simulink model "oneFingerGACTest2015a"  (R2015a)
settings: Solver=ode45  StartTime=0.0  StopTime=3  RelTol=1e-3
settings Model: CovModelRefEnable=off  Creator=Ricardo  LastModifiedBy=Ricardo
settings DataIOCC: SaveFormat=Dataset
settings HardwareCC: ProdBitPerPointer=64  ProdLargestAtomicFloat=Float  ProdIntDivRoundTo=Zero  ProdEndianess=LittleEndian  ProdHWDeviceType=Specified
settings GRTTargetCC: GeneratePreprocessorConditionals=Use local settings

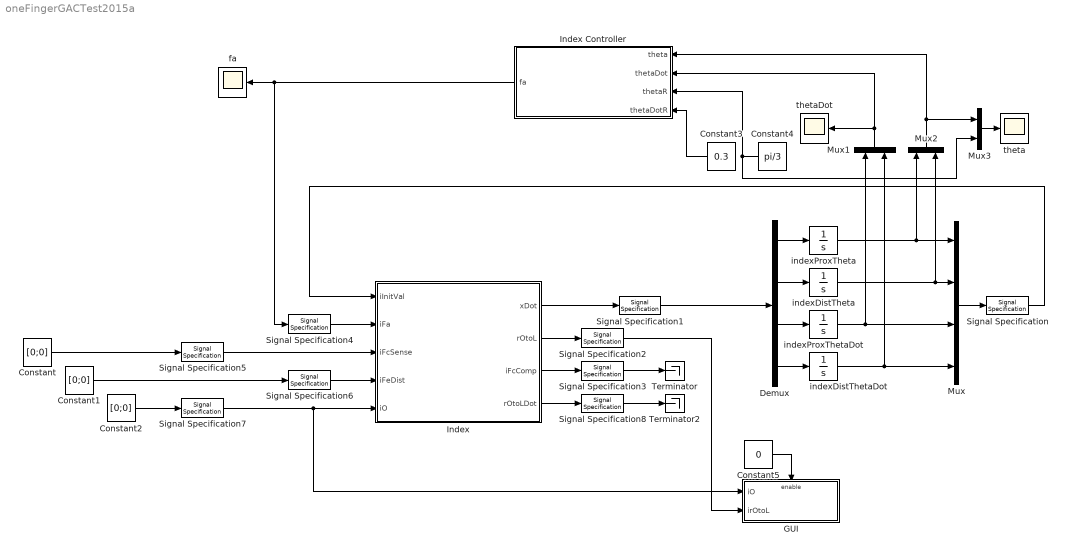
== system oneFingerGACTest2015a ==
  Constant : Constant  Value=[0;0]
  Constant1 : Constant  Value=[0;0]
  Constant2 : Constant  Value=[0;0]
  Constant3 : Constant  Value=0.3
  Constant4 : Constant  Value=pi/3
  Constant5 : Constant  Value=0
  Demux : Demux
  GUI : Subsystem  TreatAsAtomicUnit=on
  Index : MATLAB Function  TreatAsAtomicUnit=on
      settings: PermitHierarchicalResolution=ParametersOnly
  Index Controller : MATLAB Function  TreatAsAtomicUnit=on
      settings: PermitHierarchicalResolution=ParametersOnly
  Mux : Mux
  Mux1 : Mux  Inputs=2
  Mux2 : Mux  Inputs=2
  Mux3 : Mux  Inputs=2
  Signal Specification : SignalSpecification  Dimensions=4
  Signal Specification1 : SignalSpecification  Dimensions=4
  Signal Specification2 : SignalSpecification  Dimensions=[2 2]
  Signal Specification{3,5..8} (5 alike) : SignalSpecification  Dimensions=[2 1]
  Signal Specification4 : SignalSpecification  Dimensions=1
  Terminator : Terminator
  Terminator2 : Terminator
  fa : Scope
      settings: TimeRange=auto  MaxDataPoints=5000  SaveToWorkspace=off  SaveName=ScopeData2  YMin=0.78831  YMax=8.89572  SampleTime=-1
  indexDistTheta : Integrator  InitialCondition=pi/3  ContinuousStateAttributes='indexDistTheta'
  indexDistThetaDot : Integrator  ContinuousStateAttributes='indexDistThetaDot'
  indexProxTheta : Integrator  InitialCondition=pi/10  ContinuousStateAttributes='indexProxTheta'
  indexProxThetaDot : Integrator  ContinuousStateAttributes='indexProxThetaDot'
  theta : Scope
      settings: TimeRange=auto  MaxDataPoints=5000  SaveToWorkspace=off  SaveName=ScopeData3  YMin=0.20026  YMax=1.33927  SampleTime=-1
  thetaDot : Scope
      settings: TimeRange=auto  MaxDataPoints=5000  SaveToWorkspace=off  SaveName=ScopeData  YMin=-1.55545  YMax=7.74846  SampleTime=-1
  wires:
  Demux/1 -> indexProxTheta/1
  Demux/2 -> indexDistTheta/1
  Demux/3 -> indexProxThetaDot/1
  Demux/4 -> indexDistThetaDot/1
  indexProxTheta/1 -> Mux2/1, Mux/1
  indexDistTheta/1 -> Mux2/2, Mux/2
  indexProxThetaDot/1 -> Mux1/1, Mux/3
  indexDistThetaDot/1 -> Mux1/2, Mux/4
  Index/1(xDot) -> Signal Specification1/1
  Mux/1 -> Signal Specification/1
  Index/2(rOtoL) -> Signal Specification2/1
  Signal Specification/1 -> Index/1(iInitVal)
  Signal Specification1/1 -> Demux/1
  Index Controller/1(fa) -> fa/1, Signal Specification4/1
  Constant/1 -> Signal Specification5/1
  Constant1/1 -> Signal Specification6/1
  Constant2/1 -> Signal Specification7/1
  Signal Specification3/1 -> Terminator/1
  Index/3(iFcComp) -> Signal Specification3/1
  Signal Specification4/1 -> Index/2(iFa)
  Signal Specification5/1 -> Index/3(iFcSense)
  Signal Specification6/1 -> Index/4(iFeDist)
  Signal Specification8/1 -> Terminator2/1
  Index/4(rOtoLDot) -> Signal Specification8/1
  Mux2/1 -> Index Controller/1(theta), Mux3/1
  Mux1/1 -> thetaDot/1, Index Controller/2(thetaDot)
  Constant4/1 -> Index Controller/3(thetaR), Mux3/2
  Mux3/1 -> theta/1
  Signal Specification2/1 -> GUI/2(irOtoL)
  Constant3/1 -> Index Controller/4(thetaDotR)
  Signal Specification7/1 -> GUI/1(iO), Index/5(iO)
  Constant5/1 -> GUI/Enable

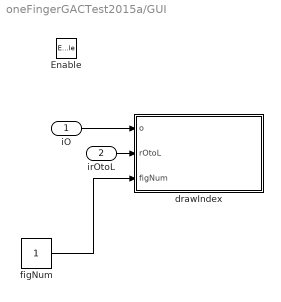
== system oneFingerGACTest2015a/GUI ==
  iO : Inport
  irOtoL : Inport  Port=2
  Enable : EnablePort
  drawIndex : MATLAB Function  TreatAsAtomicUnit=on
      settings: PermitHierarchicalResolution=ParametersOnly
  figNum : Constant
  wires:
  figNum/1 -> drawIndex/3(figNum)
  irOtoL/1 -> drawIndex/2(rOtoL)
  iO/1 -> drawIndex/1(o)

== matlab function oneFingerGACTest2015a/Index Controller ==
  data: theta input; fa output; thetaDot input; thetaR input; thetaDotR input
function fa = GAC(theta,thetaDot,thetaR,thetaDotR)
% Grasp Approach Controller
% Passivity based controller that tracks a desired approach speed.
    kP = 0.043;
    kD = 0.185;
    rP = 0.02;
    rD = 0.012;
    K = [kP 0;
         0 kD];
    Ja = [rP rD];
    theta0 = [pi/10;pi/3];
    % Reference conversion
    thetaRef = [thetaR; 0];
    thetaDotRef = [thetaDotR; 0];
% %     % Controller gains
%     Kp = [0.3, 0;
%           0, 0.3];
%     Kd = [0.01, 0;
%           0, 0.01];
%     tauA = K*(theta-theta0)-Kp*([theta(1);0]-thetaRef)-Kd*(thetaDot);
    % Controller gains
    Kp = [0, 0;
          0, 0];
    Kd = [0.08, 0;
          0, 0.08];
    tauA = K*(theta-theta0)-Kp*([theta(1);0]-thetaRef)-Kd*([thetaDot(1);0]-thetaDotRef);
%     if(tauA(1)<=0)
%         tauA(1)=0;
%     end
%     if(tauA(2)<=0)
%         tauA(2)=0;
%     end
    fa = pinv(Ja')*tauA;
end

== matlab function oneFingerGACTest2015a/Index ==
  data: iInitVal input; xDot output; iFa input; iFcSense input; iFeDist input; iO input; rOtoL output; iFcComp output; rOtoLDot output
% Finger Simulink function.
% Represents an underactuated cable driven finger.
% The finger is composed of two phalanges driven by a tendon-pulley
% mechanism. This has methods for calculating the kinematics and
% dynamics of the system.
% Author: Ricardo Garcia Rosas
% Change log:
%%%%%%%%%%%%|%%%%%%%%%%%|%%%%%%%%%%%%%%%%%%%%%%%%%%%%%%%%%%%%%%%%%%%|
% Date      |   Author  | Notes                                     |
% 16/03/23  |   RGR     | Added more comments.                      |
% 16/03/24  |   RGR     | Compute fc and transform to [x,y].        |
% 16/04/06  |   RGR     | Removed force class, using only magnitude.|
% 16/04/09  |   RGR     | Removed classes and opted for functions.  |

function [ xDot, rOtoL, iFcComp, rOtoLDot ] = Finger( iInitVal,iFa,iFcSense,iFeDist,iO )

    % Set initial condition:
    theta = [iInitVal(1); iInitVal(2)];
    thetaDot = [iInitVal(3); iInitVal(4)];
    % Transform forces:
    % Contact force
    fcTN = rotMat(theta(1,1)+theta(2,1))'*iFcSense;
    fcD = fcTN(2,1);
    if(fcD>0)
        fcD=0;
    end
    % Disturbance force
    feTN = rotMat(theta(1,1)+theta(2,1))'*iFeDist;
    feD = feTN(2,1);
    % Set model variables:
    kP = 0.043;
    kD = 0.185;
    dP = 0.01;
    dD = 0.01;
    lP = 0.1;
    lD = 0.1;
    rP = 0.02;
    rD = 0.012;
    aP = 0.1;
    aD = 0.1;
    bP = 0.05;
    bD = 0.05;
    mP = 0.02;
    mD = 0.02;
    theta0 = [pi/10;pi/3];
    IP = mP*(lP^2)/3;
    ID = mD*(lD^2)/12;
    % Set matrices
    K = [kP 0;
         0 kD];
    D = [dP 0;
         0 dD];
    Ja = [rP rD];
    Jc = [aP, 0;
          aD+lP*cos(theta(2,1)),aD];
    Je = [bP, 0;
          bD+lP*cos(theta(2,1)),bD]; 

    % Forward kinematics to link ends and centre of gravity.
    % rOtoL vector from finger origin to link end, one 2D
    % vector for each link.
    % rOtoG vector from finger origin to link center of
    % gravity, one 2D vector for each link.
    rOtoL = zeros(2,2);
    rOtoG = zeros(2,2);
    rOtoL(:,1) = iO + rotMat(theta(1,1))*[lP;0];
    rOtoG(:,1) = iO + rotMat(theta(1,1))*[lP/2;0];
    rOtoL(:,2) = rOtoL(:,2-1) + rotMat(theta(1,1)+theta(2,1))*[lD;0];
    rOtoG(:,2) = rOtoG(:,2-1) + rotMat(theta(1,1)+theta(2,1))*[lD/2;0];
    
    % Dynamics
    rOtoLDot = [-lP*sin(theta(1,1))*thetaDot(1,1)-lD*sin(theta(1,1)+theta(2,1))*(thetaDot(1,1)+thetaDot(2,1));
                -lP*cos(theta(1,1))*thetaDot(1,1)-lD*cos(theta(1,1)+theta(2,1))*(thetaDot(1,1)+thetaDot(2,1))];
    % Compute matrix parameters.
    alpha = IP + ID + (mP*(lP/2)^2) + mD*(lP^2+(lD/2)^2);
    beta = mD*lP*(lD/2);
    delta = ID+mD*(lD/2)^2;
    % Intertia matrix (M)
    M = [alpha+2*beta*cos(theta(2,1)) delta+beta*cos(theta(2,1));
         delta+beta*cos(theta(2,1)) delta];
    % Coriolis and Centrifugal matrix (C)
    C = [-beta*sin(theta(2,1))*thetaDot(2,1) ...
         -beta*sin(theta(2,1))*(thetaDot(1,1)+thetaDot(2,1));
         beta*sin(theta(2,1))*thetaDot(1,1) 0];
    % Torques
    springTau = K*(theta-theta0);
    damperTau = D*thetaDot;
    contactTau = Jc'*[0; fcD];
    distTau = Je'*[0; feD];
    actTau = Ja'*iFa;
    % Compute angular acceleration
    thetaDotDot = inv(M)*(-C*thetaDot - springTau - damperTau + contactTau + distTau + actTau);
    xDot = [thetaDot; thetaDotDot];
    % Compute applied contact force give a static condition. (Kinetostatic)
    % Compute forces normal to proximal and distal links.
    fcComp = (inv(Jc')*((springTau+damperTau)-(distTau+actTau)));
    % Distal normal and tangential (0, no tangential force due to
    % actuation) forces and transform to [x,y] coordinate.
    iFcComp = -rotMat(theta(1,1)+theta(2,1))*[0;fcComp(2,1)];
end
        function rot = rotMat(theta)
            % 2D Z-Rotation matrix on theta.
            % @param theta the angle
            % @return rot the rotation matrix as a 2x2 matrix.
            rot = [cos(theta) -sin(theta);
                   sin(theta) cos(theta)];
        end

== matlab function oneFingerGACTest2015a/GUI/drawIndex ==
  data: o input; rOtoL input; figNum input
% Plots finger to the default figure. Handled in Simulink.
% Author: Ricardo Garcia Rosas
% Change log:
%%%%%%%%%%%%|%%%%%%%%%%%|%%%%%%%%%%%%%%%%%%%%%%%%%%%%%%%%%%%%%%%%%%%|
% Date      |   Author  | Notes                                     |
% 16/03/23  |   RGR     | Added more comments.                      |
function drawFinger(o,rOtoL,figNum)
    % Plots the finger to the default figure. Handled in Simulink.
    % @param o finger origin position [x,y] (m).
    % @param rOtoL finger vector from its origin to its link
    % ends.
    % @param figNum the figure number for the plot.

    % Call figure
    figure(figNum);
    clf;
    hold on;
    % Draw Proximal components
    plot([o(1) rOtoL(1,1)],[o(2) rOtoL(2,1)],'LineWidth',8,'Color', 'k');
    plot(o(1),o(2),'ko','MarkerSize',18);
    % Draw Distal components
    plot([rOtoL(1,1) rOtoL(1,2)],[rOtoL(2,1) rOtoL(2,2)],'LineWidth',8,'Color', 'k');
    plot(rOtoL(1,1),rOtoL(2,1),'ko','MarkerSize',18);
    % Draw fingertip
    plot(rOtoL(1,2),rOtoL(2,2),'ko','MarkerSize',8);
    hold off;
    axis([-0.2 0.2 -0.05 0.2]);
end
